simulink model "SimulinkRobot_Test4_MomentumObserver"  (R2023b)
settings: Solver=VariableStepAuto  StartTime=0.0  StopTime=10  RelTol=1e-3
values from neighbouring files (symbols this model uses):
  grav = [0 0 0 0 0 -9.8]    [UR5_Data.mat]
  Mlist = [0.0102675 0 0 0 0 0 0 0.0102675 0 0 0 0 ... (216 elements, 6x6x6)]    [UR5_Data.mat]
  TfLists = [1 0 0 0 0 1 0 0 0 0 1 0 ... (112 elements, 4x4x7)]    [UR5_Data.mat]    (also in UR5_Regressor.mat)
  Twists = [xi1',xi2',xi3',xi4',xi5',xi6']    [Example1_InvKin.m]    (also in UR5_Data.mat = [0 0 1 0 0 0 0 1 0 -0.089 0 0 ... (36 elements, 6x6)]; UR5_Regressor.mat = [0 0 1 0 0 0 0 1 0 -0.089 0 0 ... (36 elements, 6x6)])
libraries: matrix_library x4, slpidlib x1
settings Model: Creator=mechmedic  LastModifiedBy=mechmedic

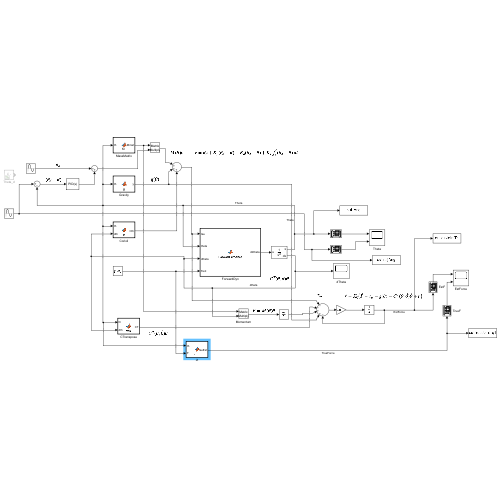
[thumbnail: Simulink's stored preview of the top-level diagram]
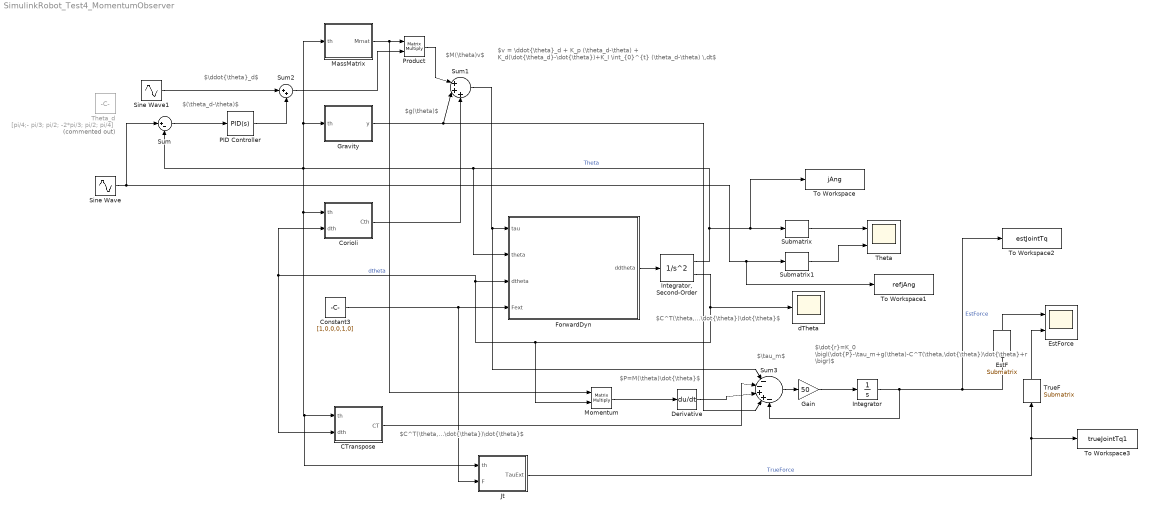
== system SimulinkRobot_Test4_MomentumObserver ==
  note: $(\theta_d-\theta)$
  note: $\ddot{\theta}_d$
  note: $g(\theta)$
  note: $C^T(\theta,\dot{\theta})\dot{\theta}$
  note: $M(\theta)v$
  note: $v = \ddot{\theta}_d + K_p (\theta_d-\theta) + K_d(\dot{\theta_d}-\dot{\theta})+K_I \int_{0}^{t} (\theta_d-\theta) \,dt$
  note: $P=M(\theta)\dot{\theta}$
  note: $\tau_m$
  note: $C^T(\theta,\dot{\theta})\dot{\theta}$
  note: $\dot{r}=K_0 \bigl(\dot{P}-\tau_m+g(\theta)-C^T(\theta,\dot{\theta})\dot{\theta}+r \bigr)$
  CTranspose : MATLAB Function  TreatAsAtomicUnit=on
  Constant3 : Constant  Value=[1,0,0,0,1,0]
  Corioli : MATLAB Function  TreatAsAtomicUnit=on
  Derivative : Derivative
  EstF : matrix_library/Submatrix  RowSpan=One row  RowStartMode=Index  RowStartIndex=5  RowEndMode=Last  RowEndIndex=1  ColSpan=All columns  ColStartMode=First  ColStartIndex=1  ColEndMode=Last  ColEndIndex=1
  EstForce : Scope  NumInputPorts=2
  ForwardDyn : MATLAB Function  TreatAsAtomicUnit=on
  Gain : Gain  Gain=50
  Gravity : MATLAB Function  TreatAsAtomicUnit=on
  Integrator : Integrator
  "Integrator, Second-Order" : SecondOrderIntegrator
  Jt : MATLAB Function  TreatAsAtomicUnit=on
  MassMatrix : MATLAB Function  TreatAsAtomicUnit=on
  Momentum : Product  Multiplication=Matrix(*)
  PID Controller : slpidlib/PID Controller  Controller=PID  Form=Parallel  TimeDomain=Continuous-time  UseExternalTs=off  SampleTime=-1  IntegratorMethod=Forward Euler  FilterMethod=Forward Euler  ControllerParametersSource=internal  P=30  I=0  UseKiTs=off  D=10  N=100  UseFilter=on  TunerSelectOption=Transfer Function Based (PID Tuner App)  InitialConditionSource=internal  InitialConditionForIntegrator=0  InitialConditionForFilter=0  DifferentiatorICPrevScaledInput=0  ExternalReset=none  TrackingMode=off  Kt=1  LimitOutput=off  SatLimitsSource=internal  UpperSaturationLimit=inf  LowerSaturationLimit=-inf  LinearizeAsGain=on  AntiWindupMode=none  Kb=1  LimitIntegrator=off  UpperIntegratorSaturationLimit=inf  LowerIntegratorSaturationLimit=-inf  POutMin=[]  POutMax=[]  IOutMin=[]  IOutMax=[]  DOutMin=[]  DOutMax=[]  NOutMin=[]  NOutMax=[]  SumOutMin=[]  SumOutMax=[]  SaturationOutMin=[]  SaturationOutMax=[]  PParamMin=[]  PParamMax=[]  IParamMin=[]  IParamMax=[]  DParamMin=[]  DParamMax=[]  NParamMin=[]  NParamMax=[]  KbParamMin=[]  KbParamMax=[]  KtParamMin=[]  KtParamMax=[]  KbOutMin=[]  KbOutMax=[]  KtOutMin=[]  KtOutMax=[]  IntegratorOutMin=[]  IntegratorOutMax=[]  FilterOutMin=[]  FilterOutMax=[]  SumI1OutMin=[]  SumI1OutMax=[]  SumI2OutMin=[]  SumI2OutMax=[]  SumI3OutMin=[]  SumI3OutMax=[]  SumI4OutMin=[]  SumI4OutMax=[]  SumDOutMin=[]  SumDOutMax=[]  DifferentiatorOutMin=[]  DifferentiatorOutMax=[]  FilterDiffOutCoefMin=[]  FilterDiffOutCoefMax=[]  ReciprocalOutMin=[]  ReciprocalOutMax=[]  SumDenOutMin=[]  SumDenOutMax=[]  SumNumOutMin=[]  SumNumOutMax=[]  DivideOutMin=[]  DivideOutMax=[]  UdiffTsProdOutMin=[]  UdiffTsProdOutMax=[]  NTsProdOutMin=[]  NTsProdOutMax=[]  UintegralTsProdOutMin=[]  UintegralTsProdOutMax=[]  UngainTsProdOutMin=[]  UngainTsProdOutMax=[]  ClampingZeroOutDataTypeStr=Inherit: Inherit via back propagation  ClampingZeroOutMin=[]  ClampingZeroOutMax=[]  FilterDenConstantOutDataTypeStr=Inherit: Inherit via back propagation  FilterDenConstantOutMin=[]  FilterDenConstantOutMax=[]  PCopyOutDataTypeStr=Inherit: Inherit via back propagation  PCopyOutMin=[]  PCopyOutMax=[]  NCopyOutDataTypeStr=Inherit: Inherit via back propagation  NCopyOutMin=[]  NCopyOutMax=[]  IntegratorContinuousStateAttributes=''  IntegratorStateMustResolveToSignalObject=off  IntegratorRTWStateStorageClass=Auto  FilterContinuousStateAttributes=''  FilterStateMustResolveToSignalObject=off  FilterRTWStateStorageClass=Auto  ParallelPVariant=InternalParameters  IdealPVariant=Disabled  IVariant=InternalParameters  DVariant=InternalParameters  IntegratorVariant=Continuous  SatVariant=Disabled  AWVariant=Passthrough  PCopyVariant=Disabled  TRVariant=Disabled  FdbkBlocksVariant=Forward  IdealPFdbkVariant=Disabled  SatFdbkVariant=Disabled  DerivativeFilterVariant=ContFilter  NVariant=InternalParameters  NCopyVariant=Disabled  FilterICVariant=InternalICsFilter  IntegratorICVariant=InternalICs  ExternalResetVariant=Disabled  TRSumVariant=Passthrough  SumFdbkVariant=Disabled  SumVariant=Sum_PID  TsampFilterVariant=InternalTs  TsampNgainVariant=Passthrough  TsampIntegralVariant=Disabled_SignalSpec  ExternalSaturationOutDataTypeStr=Inherit: Same as second input
  Product : Product  Multiplication=Matrix(*)
  Sine Wave : Sin  Amplitude=[pi/3, -pi/2, pi/3, pi/2, pi/4, pi/2]  Frequency=[1, 1, 1, 1, 1, 1]  SampleTime=0
  Sine Wave1 : Sin  Amplitude=-[pi/3, -pi/2, pi/3, pi/2, pi/4, pi/2]  Frequency=[1, 1, 1, 1, 1, 1]  SampleTime=0
  Submatrix : matrix_library/Submatrix  RowSpan=One row  RowStartMode=Index  RowStartIndex=5  RowEndMode=Last  RowEndIndex=1  ColSpan=All columns  ColStartMode=First  ColStartIndex=1  ColEndMode=Last  ColEndIndex=1
  Submatrix1 : matrix_library/Submatrix  RowSpan=One row  RowStartMode=Index  RowStartIndex=5  RowEndMode=Last  RowEndIndex=1  ColSpan=All columns  ColStartMode=First  ColStartIndex=1  ColEndMode=Last  ColEndIndex=1
  Sum : Sum  Inputs=|+-
  Sum1 : Sum  Inputs=|+++
  Sum2 : Sum  Inputs=|++
  Sum3 : Sum  Inputs=|--++-
  Theta : Scope  NumInputPorts=2
  Theta_d : Constant  Commented=on  Value=[pi/4;- pi/3; pi/2; -2*pi/3; pi/2; pi/4]
  To Workspace : ToWorkspace  VariableName=jAng  SaveFormat=Timeseries  SampleTime=-1
  To Workspace1 : ToWorkspace  VariableName=refjAng  SaveFormat=Timeseries  SampleTime=-1
  To Workspace2 : ToWorkspace  VariableName=estJointTq  SaveFormat=Timeseries  SampleTime=-1
  To Workspace3 : ToWorkspace  VariableName=trueJointTq1  SaveFormat=Timeseries  SampleTime=-1
  TrueF : matrix_library/Submatrix  RowSpan=One row  RowStartMode=Index  RowStartIndex=5  RowEndMode=Last  RowEndIndex=1  ColSpan=All columns  ColStartMode=First  ColStartIndex=1  ColEndMode=Last  ColEndIndex=1
  dTheta : Scope
  wires:
  Constant3/1 -> Jt/2(F), ForwardDyn/4(Fext)
  ForwardDyn/1(ddtheta) -> "Integrator, Second-Order"/1
  "Integrator, Second-Order"/1 -> Jt/1(th), CTranspose/1(th), Corioli/1(th), Gravity/1(th), MassMatrix/1(th), Sum/2, ForwardDyn/2(theta), To Workspace/1, Submatrix/1  "Theta"
  "Integrator, Second-Order"/2 -> dTheta/1, Momentum/2, Corioli/2(dth), CTranspose/2(dth), ForwardDyn/3(dtheta)  "dtheta"
  Gravity/1(y) -> Sum1/2, Sum3/4
  Sum/1 -> PID Controller/1
  Sum1/1 -> ForwardDyn/1(tau), Sum3/1
  Sine Wave/1 -> To Workspace1/1, Submatrix1/1, Sum/1
  PID Controller/1 -> Sum2/2
  Sum2/1 -> Product/2
  MassMatrix/1(Mmat) -> Momentum/1, Product/1
  Product/1 -> Sum1/1
  Sine Wave1/1 -> Sum2/1
  Corioli/1(Cth) -> Sum1/3
  Submatrix/1 -> Theta/1
  Submatrix1/1 -> Theta/2
  Momentum/1 -> Derivative/1
  Derivative/1 -> Sum3/3
  Sum3/1 -> Gain/1
  Integrator/1 -> To Workspace2/1, EstF/1, Sum3/5  "EstForce"
  Gain/1 -> Integrator/1
  CTranspose/1(CT) -> Sum3/2
  Jt/1(TauExt) -> To Workspace3/1, TrueF/1  "TrueForce"
  EstF/1 -> EstForce/1
  TrueF/1 -> EstForce/2

== matlab function SimulinkRobot_Test4_MomentumObserver/Gravity ==
  data: th input; y output; Twists parameter; TfLists parameter; Mlist parameter; grav parameter
function y = g(th, Twists, TfLists, Mlist, grav)
    y = GravityTorque(th, Twists, TfLists, Mlist, grav);

== matlab function SimulinkRobot_Test4_MomentumObserver/ForwardDyn ==
  settings: sampleTime=0.01
  data: tau input size=[6 1]; theta input double size=[6 1]; dtheta input double size=[6 1]; Fext input; Twists parameter size=size(Twists); TfLists parameter size=size(TfLists); ddtheta output double size=[6 1]; Mlist parameter size=size(Mlist); grav parameter size=size(grav)
function ddtheta =  ForwardDynamic (tau, theta, dtheta, Fext, Twists, TfLists, Mlist, grav)
    ddtheta =  FwdDyn(tau, theta, dtheta, Fext, Twists, TfLists, Mlist, grav);

== matlab function SimulinkRobot_Test4_MomentumObserver/MassMatrix ==
  data: th input; Mmat output; Twists parameter; TfLists parameter; Mlist parameter
function Mmat = M(th,Twists, TfLists, Mlist)
    Mmat = MassMatrix(th, Twists, TfLists, Mlist);

== matlab function SimulinkRobot_Test4_MomentumObserver/Corioli ==
  data: th input; dth input; Cth output; Twists parameter; TfLists parameter; Mlist parameter
function Cth = c(th, dth, Twists, TfLists, Mlist)
    Cth = CoriolisTorque(th, dth, Twists, TfLists, Mlist);

== matlab function SimulinkRobot_Test4_MomentumObserver/CTranspose ==
  data: th input; dth input; CT output; Twists parameter; TfLists parameter; Mlist parameter
function CT = ctth(th, dth, Twists, TfLists, Mlist)
    C = CoriolisMatrix(th,dth,Twists, TfLists, Mlist);
    CT = C'*dth;

== matlab function SimulinkRobot_Test4_MomentumObserver/Jt ==
  data: th input; F input; TauExt output; Twists parameter; TfLists parameter
function TauExt = JtF(th, F, Twists, TfLists)
    Jb = JacobianBody(th,Twists,TfLists(:,:,end));
    TauExt = Jb'*F;
